simulink model "trimNonlinearAirframe"  (R2016b)
settings: Solver=ode3  StartTime=0  StopTime=100  FixedStep=Ts  RelTol=1e-3  EnableMultiTasking=on
settings Model: Creator=The MathWorks, Inc.  LastModifiedBy=The MathWorks, Inc.
settings DataIOCC: ExternalInput=maneuverHover.getElement('Actuators'),maneuverHover.getElement('Gravity_ned'),maneuverHover.getElement('air_temp'),maneuverHover.getElement('speed_sound'),maneuverHover.getElement('pressure'),maneuverHover.getElement('air_density'),maneuverHover.getElement('MagneticField_ned')  InitialState=getstatestruct(op_trim4)  SaveFormat=StructureWithTime  SaveOutput=off  DSMLogging=off  SaveTime=off
settings OptimizationCC: BlockReduction=off  DefaultParameterBehavior=Inlined  BufferReuse=off  LifeSpan=inf
settings DebuggingCC: AlgebraicLoopMsg=none  UnderspecifiedInitializationDetection=Classic  MergeDetectMultiDrivingBlocksExec=none  UnconnectedInputMsg=none  UnconnectedOutputMsg=none  UnconnectedLineMsg=none  AllowSymbolicDim=off  SFUnexpectedBacktrackingDiag=warning  SFNoUnconditionalDefaultTransitionDiag=warning  SFExecutionAtInitializationDiag=none
settings HardwareCC: ProdBitPerPointer=32  ProdBitPerSizeT=32  ProdBitPerPtrDiffT=32  ProdLargestAtomicFloat=None  ProdIntDivRoundTo=Undefined  ProdEndianess=Unspecified  ProdWordSize=32  ProdHWDeviceType=32-bit Generic
settings ModelReferenceCC: PropagateSignalLabelsOutOfModel=off
settings GRTTargetCC: TargetLangStandard=C89/C90 (ANSI)  GeneratePreprocessorConditionals=Disable all
settings ConfigComp: CovMetricSettings=dw  CovHtmlReporting=on  CovSaveCumulativeToWorkspaceVar=on  CovSaveSingleToWorkspaceVar=on  CovExternalEMLEnable=off  CovSFcnEnable=off

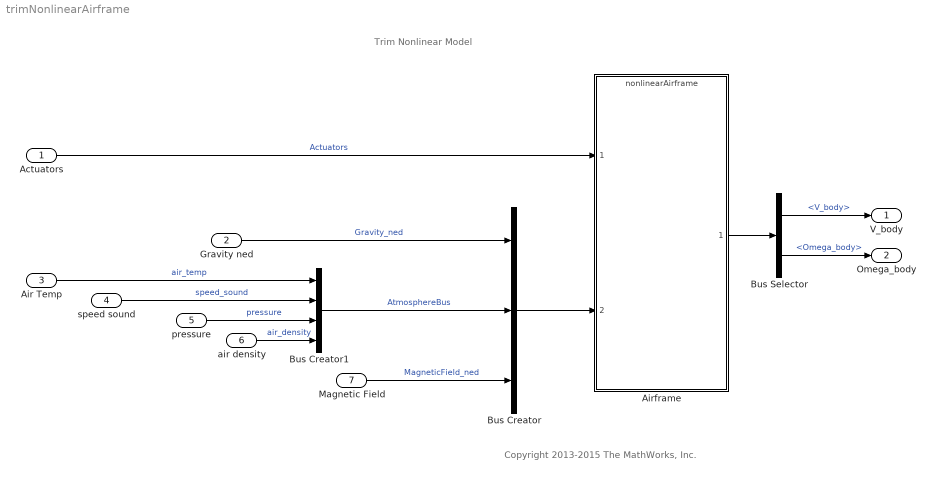
== system trimNonlinearAirframe ==
  note: Trim Nonlinear Model
  note: Copyright 2013-2015 The MathWorks, Inc.
  Actuators : Inport  PortDimensions=[1 4]
  Gravity ned : Inport  Port=2  Unit=m/s^2
  Air Temp : Inport  Port=3  Unit=K
  speed sound : Inport  Port=4  Unit=m/s
  pressure : Inport  Port=5  Unit=Pa
  air density : Inport  Port=6  Unit=kg/m^3
  Magnetic Field : Inport  Port=7  Unit=nT
  Airframe : ModelReference  ModelNameDialog=nonlinearAirframe.slx  SimulationMode=Normal  Variant=on  ModelReferenceVersion=1.97
  Bus Creator : BusCreator  Inputs=3  OutDataTypeStr=Bus: EnvironmentBus  NonVirtualBus=on
  Bus Creator1 : BusCreator  Inputs=4  OutDataTypeStr=Bus: AtmosphereBus  NonVirtualBus=on
  Bus Selector : BusSelector  OutputSignals=V_body,Omega_body
  V_body : Outport  Unit=m/s
  Omega_body : Outport  Port=2  Unit=rad/s
  wires:
  Actuators/1 -> Airframe/1  "Actuators"
  Airframe/1 -> Bus Selector/1
  Magnetic Field/1 -> Bus Creator/3  "MagneticField_ned"
  Bus Creator1/1 -> Bus Creator/2  "AtmosphereBus"
  air density/1 -> Bus Creator1/4  "air_density"
  pressure/1 -> Bus Creator1/3  "pressure"
  speed sound/1 -> Bus Creator1/2  "speed_sound"
  Air Temp/1 -> Bus Creator1/1  "air_temp"
  Bus Creator/1 -> Airframe/2
  Gravity ned/1 -> Bus Creator/1  "Gravity_ned"
  Bus Selector/1 -> V_body/1  "<V_body>"
  Bus Selector/2 -> Omega_body/1  "<Omega_body>"
